simulink library "xbsDSP_r4"  (Simulink 7.1)
PreLoadFcn:
  | warning('off','MATLAB:mex:deprecatedExtension');xlmeta;com.xilinx.sysgen.util.StrategyUtil.loadAllStrategyNames();
undefined symbols (not defined in the file or in its folder): A, A2, B, C, D, gcbh, X, xlBlockLoadCallback, xlipgetpartsetting, Z
libraries: xbsIndex_r4 x27
settings Model: Tag=SysGenIndex  Creator=sysgengroup  LastModifiedBy=sysgengroup

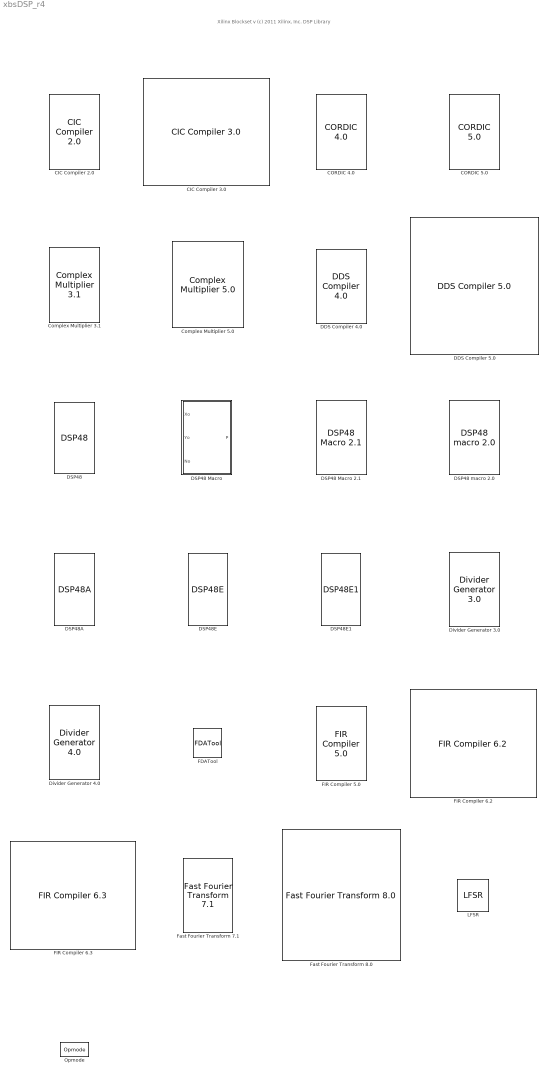
== system xbsDSP_r4 ==
  note: Xilinx Blockset v
      | (c) 2011 Xilinx, Inc.
      |
      | DSP Library
  "CIC Compiler 2.0 " : xbsIndex_r4/CIC Compiler 2.0   filter_type=Interpolation  number_of_stages=3  differential_delay=1  number_of_channels=1  sample_rate_changes=Fixed  fixed_or_initial_rate=4  minimum_rate=4  maximum_rate=4  ratespecification=Maximum_Possible  sampleperiod=4  hardwareoversamplingrate=1  quantization=Full_Precision  output_data_width=18  use_xtreme_dsp_slice=on  use_streaming_interface=on  sclr=off  ce=off  gui_behaviour=Sysgen  input_data_width=18  ip_name=CIC Compiler  ip_version=2.0  dsptool_ready=true  wrapper_available=true  port_translation_map={ 'ce' => 'en', 'sclr' => 'rst' }  ipcore_xco_need_fpga_part=true  ipcore_fpga_part=xlipgetpartsetting(gcb, {'virtex4', 'xc4vsx35', '-10', 'ff668'})  ipcore_verbose=false  block_type=cic_compiler_v2_0
  "CIC Compiler 3.0 " : xbsIndex_r4/CIC Compiler 3.0   filter_type=Interpolation  number_of_stages=3  differential_delay=1  number_of_channels=1  sample_rate_changes=Fixed  fixed_or_initial_rate=4  minimum_rate=4  maximum_rate=4  ratespecification=Maximum_Possible  sampleperiod=4  hardwareoversamplingrate=1  quantization=Full_Precision  output_data_width=22  use_xtreme_dsp_slice=on  use_streaming_interface=on  has_aclken=off  has_aresetn=off  has_dout_tready=off  trim_axipin_name=on  gui_behaviour=Sysgen_GUI  input_data_width=18  ip_name=CIC Compiler  ip_version=3.0  dsptool_ready=true  wrapper_available=true  port_translation_map={ 'aclken' => 'en', 'aresetn' => 'rst' }  ipcore_xco_need_fpga_part=true  ipcore_fpga_part=xlipgetpartsetting(gcb, {'virtex7', 'xc7v1500t', '-2', 'fhg1157'})  ipcore_verbose=false  block_type=cic_compiler_v3_0
  "CORDIC 4.0 " : xbsIndex_r4/CORDIC 4.0   functional_selection=Square_Root  architectural_configuration=Parallel  pipelining_mode=Maximum  data_format=UnsignedFraction  phase_format=Radians  output_width=16  round_mode=Truncate  iterations=0  precision=0  coarse_rotation=on  compensation_scaling=No_Scale_Compensation  ce=off  sclr=off  nd=off  rdy=off  x_out=on  y_out=on  phase_output=off  register_inputs=true  register_outputs=true  ipcore_usecache=true  ipcore_useipmodelcache=true  ipcore_verbose=false  wrapper_available=true  ip_name=CORDIC  ip_version=4.0  dsptool_ready=true  port_translation_map={ 'ce' => 'en', 'sclr' => 'rst' }  structural_sim=false  block_type=cordic_v4_0
  "CORDIC 5.0 " : xbsIndex_r4/CORDIC 5.0   functional_selection=Rotate  architectural_configuration=Parallel  pipelining_mode=Maximum  data_format=SignedFraction  phase_format=Radians  input_width=16  output_width=16  round_mode=Truncate  iterations=0  precision=0  compensation_scaling=No_Scale_Compensation  coarse_rotation=on  aclken=off  aresetn=off  out_tready=off  cartesian_has_tuser=off  cartesian_has_tlast=off  cartesian_tuser_width=1  phase_has_tuser=off  phase_has_tlast=off  phase_tuser_width=1  out_tlast_behv=Null  flow_control=NonBlocking  optimize_goal=Resources  trim_axipin_name=on  ip_name=CORDIC  ip_version=5.0  dsptool_ready=true  ipcore_usecache=true  ipcore_useipmodelcache=true  wrapper_available=true  port_translation_map={ 'aclken' => 'en', 'aresetn' => 'rst' }  block_type=cordic_v5_0
      settings: infoedit=CORDIC 5.0
  "Complex Multiplier 3.1 " : xbsIndex_r4/Complex Multiplier 3.1   multtype=Use_Mults  optimizegoal=Resources  outputwidthhigh=32  outputwidthlow=0  latency=-1  roundmode=Truncate  clockenable=off  syncclear=off  ip_name=Complex Multiplier  ip_version=3.1  dsptool_ready=true  ipcore_usecache=true  ipcore_useipmodelcache=true  ipcore_verbose=false  ipcore_latency_parameter='latency'  wrapper_available=true  port_translation_map={ 'ce' => 'en', 'sclr' => 'rst' }  structural_sim=false  block_type=cmpy_v3_1
  "Complex Multiplier 5.0 " : xbsIndex_r4/Complex Multiplier 5.0   hasatlast=off  hasatuser=off  atuserwidth=1  hasbtlast=off  hasbtuser=off  btuserwidth=1  multtype=Use_Mults  optimizegoal=Resources  flowcontrol=NonBlocking  outputwidth=33  roundmode=Truncate  hasctrltlast=off  hasctrltuser=off  ctrltuserwidth=1  outtlastbehv=Null  latencyconfig=Automatic  minimumlatency=15  aclken=off  aresetn=off  trim_axipin_name=on  aportwidth=63  bportwidth=63  ip_name=Complex Multiplier  ip_version=5.0  dsptool_ready=true  ipcore_usecache=true  ipcore_useipmodelcache=true  ipcore_verbose=false  ipcore_latency_parameter='minimumlatency'  wrapper_available=true  port_translation_map={ 'aclken' => 'en', 'aresetn' => 'rst'}  structural_sim=false  block_type=cmpy_v5_0
  "DDS Compiler 4.0 " : xbsIndex_r4/DDS Compiler 4.0   partspresent=Phase_Generator_and_SIN_COS_LUT  dds_clock_rate=100  channels=1  parameter_entry=System_Parameters  spurious_free_dynamic_range=36  frequency_resolution=0.4  noise_shaping=None  phase_width=28  output_width=6  output_selection=Sine_and_Cosine  negative_sine=off  negative_cosine=off  amplitude_mode=Full_Range  memory_type=Auto  optimization_goal=Auto  dsp48_use=Minimal  latency_configuration=Auto  latency=1  has_phase_out=on  sclr_pin=off  clock_enable=off  rfd=off  rdy=off  channel_pin=off  explicit_period=off  period=1  phase_increment=Fixed  output_frequency1=0  output_frequency2=0  output_frequency3=0  output_frequency4=0  output_frequency5=0  output_frequency6=0  output_frequency7=0  output_frequency8=0  output_frequency9=0  output_frequency10=0  output_frequency11=0  output_frequency12=0  output_frequency13=0  output_frequency14=0  output_frequency15=0  output_frequency16=0  pinc1='0'  pinc2='0'  pinc3='0'  pinc4='0'  pinc5='0'  pinc6='0'  pinc7='0'  pinc8='0'  pinc9='0'  pinc10='0'  pinc11='0'  pinc12='0'  pinc13='0'  pinc14='0'  pinc15='0'  pinc16='0'  phase_offset=None  phase_offset_angles1=0  phase_offset_angles2=0  phase_offset_angles3=0  phase_offset_angles4=0  phase_offset_angles5=0  phase_offset_angles6=0  phase_offset_angles7=0  phase_offset_angles8=0  phase_offset_angles9=0  phase_offset_angles10=0  phase_offset_angles11=0  phase_offset_angles12=0  phase_offset_angles13=0  phase_offset_angles14=0  phase_offset_angles15=0  phase_offset_angles16=0  poff1='0'  poff2='0'  poff3='0'  poff4='0'  poff5='0'  poff6='0'  poff7='0'  poff8='0'  poff9='0'  poff10='0'  poff11='0'  poff12='0'  poff13='0'  poff14='0'  poff15='0'  poff16='0'  por_mode=false  gui_behaviour=Sysgen  ip_name=DDS Compiler  ip_version=4.0  dsptool_ready=true  wrapper_available=true  port_translation_map={ 'ce' => 'en', 'sclr' => 'rst' }  ipcore_xco_need_fpga_part=true  ipcore_fpga_part=xlipgetpartsetting(gcb, {'virtex4', 'xc4vsx35', '-10', 'ff668'})  ipcore_usecache=true  ipcore_useipmodelcache=true  ipcore_verbose=false  block_type=dds_compiler_v4_0
  "DDS Compiler 5.0 " : xbsIndex_r4/DDS Compiler 5.0   partspresent=Phase_Generator_and_SIN_COS_LUT  dds_clock_rate=100  channels=1  parameter_entry=System_Parameters  spurious_free_dynamic_range=36  frequency_resolution=0.4  noise_shaping=None  phase_width=28  output_width=6  output_selection=Sine_and_Cosine  negative_sine=off  negative_cosine=off  amplitude_mode=Full_Range  memory_type=Auto  optimization_goal=Auto  dsp48_use=Minimal  latency_configuration=Auto  latency=1  has_phase_out=on  has_aclken=off  has_aresetn=off  explicit_period=off  period=1  data_has_tlast=Not_Required  has_tready=on  s_phase_has_tuser=Not_Required  m_data_has_tuser=Not_Required  m_phase_has_tuser=Not_Required  s_phase_tuser_width=1  s_config_sync_mode=On_Vector  phase_increment=Fixed  output_frequency1=0  output_frequency2=0  output_frequency3=0  output_frequency4=0  output_frequency5=0  output_frequency6=0  output_frequency7=0  output_frequency8=0  output_frequency9=0  output_frequency10=0  output_frequency11=0  output_frequency12=0  output_frequency13=0  output_frequency14=0  output_frequency15=0  output_frequency16=0  pinc1='0'  pinc2='0'  pinc3='0'  pinc4='0'  pinc5='0'  pinc6='0'  pinc7='0'  pinc8='0'  pinc9='0'  pinc10='0'  pinc11='0'  pinc12='0'  pinc13='0'  pinc14='0'  pinc15='0'  pinc16='0'  phase_offset=None  phase_offset_angles1=0  phase_offset_angles2=0  phase_offset_angles3=0  phase_offset_angles4=0  phase_offset_angles5=0  phase_offset_angles6=0  phase_offset_angles7=0  phase_offset_angles8=0  phase_offset_angles9=0  phase_offset_angles10=0  phase_offset_angles11=0  phase_offset_angles12=0  phase_offset_angles13=0  phase_offset_angles14=0  phase_offset_angles15=0  phase_offset_angles16=0  poff1='0'  poff2='0'  poff3='0'  poff4='0'  poff5='0'  poff6='0'  poff7='0'  poff8='0'  poff9='0'  poff10='0'  poff11='0'  poff12='0'  poff13='0'  poff14='0'  poff15='0'  poff16='0'  trim_axipin_name=on  por_mode=false  gui_behaviour=Sysgen  ip_name=DDS Compiler  ip_version=5.0  dsptool_ready=true  wrapper_available=true  port_translation_map={ 'aclken' => 'en', 'aresetn' => 'rst' }  ipcore_xco_need_fpga_part=true  ipcore_fpga_part=xlipgetpartsetting(gcb, {'virtex6', 'xc6vlx75t', '-3', 'ff784'})  ipcore_usecache=true  ipcore_useipmodelcache=true  ipcore_verbose=false  block_type=dds_compiler_v5_0
  DSP48 : xbsIndex_r4/DSP48  use_b=Direct from B Port  use_op=off  use_creg=off  use_pcin=off  use_pcout=off  use_bcout=off  rst_all=off  en_all=off  pipeline_a=1  pipeline_b=1  pipeline_c=on  pipeline_p=on  pipeline_mult=on  pipeline_opmode=on  pipeline_sub=on  pipeline_carryin=on  pipeline_carryinsel=on  rst_a=off  rst_b=off  rst_c=off  rst_mult=off  rst_p=off  rst_carry_in=off  rst_ctrl=off  en_a=off  en_b=off  en_c=off  en_mult=off  en_p=off  en_carry_in=off  en_ctrl=off  dbl_ovrd=off  use_synth_model=off  xl_useadderonly=off  block_type=dsp48
  DSP48 Macro : Subsystem  LoadFcn=xlBlockLoadCallback(gcbh);  mask(Xilinx DSP48 Macro Block){infoedit=Macro function to simplify use of the DSP48 primitive, especially as a dynamic operator, portalist=Xo, portblist=Yo, portclist=No, instrlist=|, pipeline_sgadvanced=, pipeline=Custom, pipeachoices_sgadvanced=, pipeachoices=1, pipebchoices_sgadvanced=, pipebchoices=1, pipecchoices_sgadvanced=, pipecchoices=on, pipepchoices_sgadvanced=, pipepchoices=on, pipemchoices_sgadvanced=, pipemchoices=on, pipectrlchoices_sgadvanced=, pipectrlchoices=on, pipemuxachoices_sgadvanced=, pipemuxachoices=0, pipemuxbchoices_sgadvanced=, pipemuxbchoices=0, pipemuxcchoices_sgadvanced=, pipemuxcchoices=0, pipemuxctrlchoices_sgadvanced=, pipemuxctrlchoices=0, pipeline_array_flag_sgadvanced=, pipeline_array_flag=off, custom_pipeline_cache=[1  1  1  1  1  1  0  0  0  0], precision_sgadvanced=, precision=Full, arith_type_sgadvanced=, arith_type=Unsigned, n_bits=8, bin_pt=2, bcout_sgadvanced=, bcout=off, acout_sgadvanced=, acout=off, carryout_sgadvanced=, carryout=off, carrycascout_sgadvanced=, carrycascout=off, pcout_sgadvanced=, pcout=off, rst_all_sgadvanced=, rst_all=off, rst_a_sgadvanced=, rst_a=off, rst_b_sgadvanced=, rst_b=off, rst_c_sgadvanced=, rst_c=off, rst_m_sgadvanced=, rst_m=off, rst_p_sgadvanced=, rst_p=off, rst_ctrl_sgadvanced=, rst_ctrl=off, ce_all_sgadvanced=, ce_all=off, ce_a_sgadvanced=, ce_a=off, ce_b_sgadvanced=, ce_b=off, ce_c_sgadvanced=, ce_c=off, ce_m_sgadvanced=, ce_m=off, ce_p_sgadvanced=, ce_p=off, ce_ctrl_sgadvanced=, ce_ctrl=off, dbl_ovrd_sgadvanced=, dbl_ovrd=off, synth_opt_sgadvanced=, synth_opt=on, errorlist=false, statestr=2d82c218ef9225b6e0048b8063710b3c, explicit_period=, period=1, maskdoc=, has_advanced_control=0, sggui_pos=-1,-1,-1,-1, block_type=dsp48macro, block_version=8.2.1, sg_icon_stat=90,138,3,1,white,blue,0,024d3c91cd129fc3834d91e223da5447,right,,[ ],[ ], sg_mask_display=|, sg_list_contents=, sg_blockgui_xml=}
      mask instrlist=|
      | <html><head><meta name="qrichtext" content="1" /></head><body style="font-size:8pt;font-family:MS Shell Dlg">
      | <p>P=Xo*Yo+No</p>
      | </body></html>
      mask sg_mask_display=|
      | fprintf('','COMMENT: begin icon graphics');
      | patch([0 90 90 0 0 ],[0 0 138 138 0 ],[0.77 0.82 0.91 ]);
      | plot([0 90 90 0 0 ],[0 0 138 138 0 ]);
      | patch([18.3 35.64 47.64 59.64 71.64 47.64 30.3 18.3 ],[82.32 82.32 94.32 82.32 94.32 94.32 94.32 82.32 ],[1 1 1 ]);
      | patch([30.3 47.64 35.64 18.3 30.3 ],[70.32 70.32 82.32 82.32 70.32 ],[0.931 0.946 0.973 ]);
      | patch([18.3 35.64 47.64 30.3 18.3 ],[58.32 58.32 70.32 70.32 58.32 ],[1 1 1 ]);
      | patch([30.3 71.64 59.64 47.64 35.64 18.3 30.3 ],[46.32 46.32 58.32 46.32 58.32 58.32 46.32 ],[0.931 0.946 0.973 ]);
      | fprintf('','COMMENT: end icon graphics');
      | fprintf('','COMMENT: begin icon text');
      | color('black');port_label('input',1,'Xo');
      | color('black');port_label('input',2,'Yo');
      | color('black');port_label('input',3,'No');
      | color('black');port_label('output',1,'P');
      | fprintf('','COMMENT: end icon text');
      mask prompts: infoedit ""; portalist "Inputs to port <tt>A</tt>"; portblist "Inputs to port <tt>B</tt>"; portclist "Inputs to port <tt>C</tt>"; instrlist "Instructions"; pipeline_sgadvanced ""; pipeline "Pipeline options"; pipeachoices_sgadvanced ""; pipeachoices "<tt>A</tt>"; pipebchoices_sgadvanced ""; pipebchoices "<tt>B</tt>"; pipecchoices_sgadvanced ""; pipecchoices "<tt>C</tt>"; pipepchoices_sgadvanced ""; pipepchoices "<tt>P</tt>"; pipemchoices_sgadvanced ""; pipemchoices "Multiplier"; pipectrlchoices_sgadvanced ""; pipectrlchoices "Controls (<tt>opmode</tt>, <tt>subtract</tt>,<br> <tt>carry_in</tt>, <tt>carry_in_sel</tt>)"; pipemuxachoices_sgadvanced ""; pipemuxachoices "MuxA"; pipemuxbchoices_sgadvanced ""; pipemuxbchoices "MuxB"; pipemuxcchoices_sgadvanced ""; pipemuxcchoices "MuxC"; pipemuxctrlchoices_sgadvanced ""; pipemuxctrlchoices "MuxCtrl"; pipeline_array_flag_sgadvanced ""; pipeline_array_flag "Define Using Array"; custom_pipeline_cache "Custom Pipeline Options([A,B,C,P,Ctrl,M,MuxA,MuxB,MuxC,MuxCtrl])"; precision_sgadvanced ""; arith_type_sgadvanced ""; arith_type "Output type"; n_bits "Number of bits"; bin_pt "Binary point"; bcout_sgadvanced ""; bcout "<tt>BCOUT</tt>"; acout_sgadvanced ""; acout "<tt>ACOUT</tt>"; carryout_sgadvanced ""; carryout "<tt>CARRYOUT</tt>"; carrycascout_sgadvanced ""; carrycascout "<tt>CARRYCASCOUT</tt>"; pcout_sgadvanced ""; pcout "<tt>PCOUT</tt>"; rst_all_sgadvanced ""; rst_all "<tt>Global Reset</tt>"; rst_a_sgadvanced ""; rst_a "Reset port for <tt>A</tt>"; rst_b_sgadvanced ""; rst_b "Reset port for <tt>B</tt>"; rst_c_sgadvanced ""; rst_c "Reset port for <tt>C</tt>"; rst_m_sgadvanced ""; rst_m "Reset port for multiplier"; rst_p_sgadvanced ""; rst_p "Reset port for <tt>P</tt>"; rst_ctrl_sgadvanced ""; rst_ctrl "Reset port for controls <br> (<tt>opmode</tt>, <tt>subtract</tt>,<br> <tt>carry_in</tt>, <tt>carry_in_sel</tt>)"; ce_all_sgadvanced ""; ce_all "<tt>Global Enable</tt>"; ce_a_sgadvanced ""; ce_a "Enable port for <tt>A</tt>"; ce_b_sgadvanced ""; ce_b "Enable port for <tt>B</tt>"; ce_c_sgadvanced ""; ce_c "Enable port for <tt>C</tt>"; ce_m_sgadvanced ""; ce_m "Enable port for multiplier"; ce_p_sgadvanced ""; ce_p "Enable port for <tt>P</tt>"; ce_ctrl_sgadvanced ""; ce_ctrl "Enable port for controls <br> (<tt>opmode</tt>, <tt>subtract</tt>,<br> <tt>carry_in</tt>, <tt>carry_in_sel</tt>)"; dbl_ovrd_sgadvanced ""; dbl_ovrd "Override with doubles"; synth_opt_sgadvanced ""; synth_opt "Use DSP48"; errorlist ""; statestr ""; explicit_period ""; period ""; maskdoc ""; has_advanced_control ""; sggui_pos ""; block_type ""; block_version ""; sg_icon_stat ""; sg_mask_display ""; sg_list_contents ""; sg_blockgui_xml ""
      mask help: Macro function to simplify use of the DSP48 primitive, especially as a dynamic operator
      mask init:
      | try
      |   tmp_gcb = gcb;
      |   tmp_gcbh = gcbh;
      |   if (strcmp('SysGenIndex',get_param(bdroot(tmp_gcbh),'tag')) && ~isempty(regexp(bdroot(tmp_gcb), '^xbs', 'once')))
      |     return;
      |   end;
      |   xlMungeMaskParams;
      | 
      |   block_type='dsp48macro';
      | 
      |   serialized_declarations = '{''block_type''=>''String''}';
      |   xldsp48macro_init();
      |   ptable_ = xlblockprep(get_param(tmp_gcb, 'MaskWSVariables'));
      |   try
      |     xlBlockMoveCallback(tmp_gcbh);
      |   catch 
      |      clear global xl_updateicon_recursion_guard;
      |   end;
      | catch
      |   global dbgsysgen;
      |   if(~isempty(dbgsysgen) && dbgsysgen)
      |     e = regexprep(lasterr, '\n', '\nError: ');
      |     disp(['Error: While running MaskInit code on block ' tmp_gcb ': ' e]);
      |     error(e);
      |   end
      | end
      settings: CopyFcn=tmp_gcbh = gcbh;set_param(tmp_gcbh,'linkstatus','none');xlBlockMoveCallback(gcbh);  DeleteFcn=xlDestroyGui(gcbh);  ModelCloseFcn=xlDestroyGui(gcbh);  PreSaveFcn=xlBlockPreSaveCallback(gcbh);  PostSaveFcn=xlBlockPostSaveCallback(gcbh);  DestroyFcn=xlDestroyGui(gcbh);  OpenFcn=xlOpenGui(gcbh, 'dsp48macro_gui.xml', @dsp48macroenablement, @dsp48macroaction)  CloseFcn=xlDestroyGui(gcbh);  MoveFcn=xlBlockMoveCallback(gcbh);
      mask Help: eval('');xlDoc('-book','sysgen','-topic','DSP48_Macro');
      mask StyleString: edit,edit,edit,edit,edit,edit,popup(External Registers|No External Registers|Custom),edit,popup(0|1|2),edit,popup(0|1|2),edit,checkbox,edit,checkbox,edit,checkbox,edit,checkbox,edit,popup(0|1|2),edit,popup(0|1|2),edit,popup(0|1|2),edit,popup(0|1|2),edit,checkbox,edit,edit,popup(Full|User Defined),edit,popup(Signed  (2's comp)|Unsigned),edit,edit,edit,checkbox,edit,checkbox,edit,checkbox,edit,checkbox,edit,checkbox,edit,checkbox,edit,checkbox,edit,checkbox,edit,checkbox,edit,checkbox,edit,checkbox,edit,checkbox,edit,checkbox,edit,checkbox,edit,checkbox,edit,checkbox,edit,checkbox,edit,checkbox,edit,checkbox,edit,checkbox,edit,checkbox,edit,edit,edit,edit,edit,edit,edit,edit,edit,edit,edit,edit,edit
      mask Display:
      | fprintf('','COMMENT: begin icon graphics');
      | patch([0 90 90 0 0 ],[0 0 138 138 0 ],[0.77 0.82 0.91 ]);
      | plot([0 90 90 0 0 ],[0 0 138 138 0 ]);
      | patch([18.3 35.64 47.64 59.64 71.64 47.64 30.3 18.3 ],[82.32 82.32 94.32 82.32 94.32 94.32 94.32 82.32 ],[1 1 1 ]);
      | patch([30.3 47.64 35.64 18.3 30.3 ],[70.32 70.32 82.32 82.32 70.32 ],[0.931 0.946 0.973 ]);
      | patch([18.3 35.64 47.64 30.3 18.3 ],[58.32 58.32 70.32 70.32 58.32 ],[1 1 1 ]);
      | patch([30.3 71.64 59.64 47.64 35.64 18.3 30.3 ],[46.32 46.32 58.32 46.32 58.32 58.32 46.32 ],[0.931 0.946 0.973 ]);
      | fprintf('','COMMENT: end icon graphics');
      | fprintf('','COMMENT: begin icon text');
      | color('black');port_label('input',1,'Xo');
      | color('black');port_label('input',2,'Yo');
      | color('black');port_label('input',3,'No');
      | color('black');port_label('output',1,'P');
      | fprintf('','COMMENT: end icon text');
  "DSP48 Macro 2.1 " : xbsIndex_r4/DSP48 Macro 2.1   instruction_list=A*B+C  AvailableInstructions=A*B+C  show_filtered=off  pipeline_options=Automatic  dspimage="<html><img src=\"xbip_dsp48_macro_v2_1_regimag.png\"></html>"  tier_1=off  tier_2=off  tier_3=off  tier_4=off  tier_5=off  tier_6=off  dreg_1=off  dreg_2=off  dreg_3=off  areg_1=off  areg_2=off  areg_3=off  areg_4=off  breg_1=off  breg_2=off  breg_3=off  breg_4=off  mreg_5=off  concatreg_3=off  concatreg_4=off  concatreg_5=off  creg_1=off  creg_2=off  creg_3=off  creg_4=off  creg_5=off  preg_6=off  cinreg_1=off  cinreg_2=off  cinreg_3=off  cinreg_4=off  cinreg_5=off  opreg_1=off  opreg_2=off  opreg_3=off  opreg_4=off  opreg_5=off  output_properties=Full_Precision  p_width=48  p_binarywidth=0  has_acout=off  has_bcout=off  has_pcout=off  has_carryout=off  has_carrycascout=off  has_ce=off  has_d_ce=off  has_a_ce=off  has_b_ce=off  has_concat_ce=off  has_c_ce=off  has_m_ce=off  has_p_ce=off  has_sel_ce=off  has_sclr=off  has_d_sclr=off  has_a_sclr=off  has_b_sclr=off  has_concat_sclr=off  has_c_sclr=off  has_m_sclr=off  has_p_sclr=off  has_sel_sclr=off  use_dsp48=on  gui_behaviour=Sysgen  instruction1=#  ip_name=DSP48 Macro  ip_version=2.1  dsptool_ready=true  ipcore_usecache=true  ipcore_useipmodelcache=true  wrapper_available=true  port_translation_map={ 'ce' => 'en', 'sclr' => 'rst'}  ipcore_xco_need_fpga_part=true  ipcore_fpga_part=xlipgetpartsetting(gcb, {'virtex6', 'xc6vlx75t', '-3', 'ff784'})  ipcore_latency_function='has_combinational'  structural_sim=false  ipcore_verbose=false  ipcore_port_config={ 'carryin' => { 'arith' => 'ufix', 'binpt' => 0.00000000000, 'width' => 1.00000000000}, 'carrycascin' => { 'arith' => 'ufix', 'binpt' => 0.00000000000, 'width' => 1.00000000000}, 'carrycascout' => { 'arith' => 'ufix', 'binpt' => 0.00000000000, 'width' => 1.00000000000}, 'carryout' => { 'arith' => 'ufix', 'binpt' => 0.00000000000, 'width' => 1.00000000000}}  block_type=xbip_dsp48_macro_v2_1
      settings: infoedit=<html>Valid operands: CONCAT, P, C, PCIN, P>>17, PCIN>>17, CARRYIN, CARRYCASCIN, ACIN, A, BCIN,B<br><br>Valid operators: +, -, *, ()<br><br>Valid functions: RNDSIMPLE, RNDSYM<br><br>Instructions are case insensitive and tolerate spaces.</html>
  "DSP48 macro 2.0 " : xbsIndex_r4/DSP48 macro 2.0   instruction_list=A*B+C  AvailableInstructions=A*B+C  show_filtered=off  pipeline_options=Automatic  dspimage="<html><img src=\"xbip_dsp48_macro_v2_0_regimag.png\"></html>"  tier_1=off  tier_2=off  tier_3=off  tier_4=off  tier_5=off  tier_6=off  dreg_1=off  dreg_2=off  dreg_3=off  areg_1=off  areg_2=off  areg_3=off  areg_4=off  breg_1=off  breg_2=off  breg_3=off  breg_4=off  mreg_5=off  concatreg_3=off  concatreg_4=off  concatreg_5=off  creg_1=off  creg_2=off  creg_3=off  creg_4=off  creg_5=off  preg_6=off  cinreg_1=off  cinreg_2=off  cinreg_3=off  cinreg_4=off  cinreg_5=off  opreg_1=off  opreg_2=off  opreg_3=off  opreg_4=off  opreg_5=off  output_properties=Full_Precision  p_width=48  p_binarywidth=0  has_carryout=off  has_acout=off  has_bcout=off  has_carrycascout=off  has_pcout=off  has_ce=off  has_sclr=off  use_dsp48=on  gui_behaviour=Sysgen  instruction1=#  ip_name=DSP48 macro  ip_version=2.0  dsptool_ready=true  ipcore_usecache=true  ipcore_useipmodelcache=true  wrapper_available=true  port_translation_map={ 'ce' => 'en', 'sclr' => 'rst'}  ipcore_xco_need_fpga_part=true  ipcore_fpga_part=xlipgetpartsetting(gcb, {'virtex4', 'xc4vsx35', '-10', 'ff668'})  ipcore_latency_function='has_combinational'  structural_sim=false  ipcore_verbose=false  ipcore_port_config={ 'carryin' => { 'arith' => 'ufix', 'binpt' => 0.00000000000, 'width' => 1.00000000000}, 'carrycascin' => { 'arith' => 'ufix', 'binpt' => 0.00000000000, 'width' => 1.00000000000}, 'carrycascout' => { 'arith' => 'ufix', 'binpt' => 0.00000000000, 'width' => 1.00000000000}, 'carryout' => { 'arith' => 'ufix', 'binpt' => 0.00000000000, 'width' => 1.00000000000}}  block_type=xbip_dsp48_macro_v2_0
      settings: infoedit=<html>Valid operands: CONCAT, P, C, PCIN, P>>17, PCIN>>17, CARRYIN, CARRYCASCIN, ACIN, A, BCIN,B<br><br>Valid operators: +, -, *, ()<br><br>Valid functions: RNDSIMPLE, RNDSYM<br><br>Instructions are case insensitive and tolerate spaces.</html>
  DSP48A : xbsIndex_r4/DSP48A  use_op=on  use_creg=off  use_d=off  use_pcin=off  use_pcout=off  use_bcout=off  use_carryin=off  use_carryout=off  rst_all=off  en_all=off  carryin_type=Direct from carry in port  use_a0reg=on  use_a1reg=on  use_b0reg=on  use_b1reg=on  pipeline_c=on  pipeline_d=on  pipeline_mult=on  pipeline_p=on  pipeline_opmode=on  pipeline_carryin=on  rst_a=off  rst_b=off  rst_c=off  rst_d=off  rst_mult=off  rst_p=off  rst_opmode=off  rst_carry_in=off  en_a=off  en_b=off  en_c=off  en_d=off  en_mult=off  en_p=off  en_opmode=off  en_carry_in=off  dbl_ovrd=off  use_synth_model=off  device=3  block_type=dsp48a
  DSP48E : xbsIndex_r4/DSP48E  use_a=Direct from A Port  use_b=Direct from B Port  reset_preg=off  pattern_from_creg=on  pattern='000000000000'  mask_from_creg=on  pattern_mask='000000000000'  sel_rounding_mask=Select mask  use_op=off  use_creg=off  rst_all=off  en_all=off  use_pcin=off  use_carrycascin=off  use_multsignin=off  use_carryout=off  use_patterndetect=off  use_patternbdetect=off  use_overflow=off  use_underflow=off  use_acout=off  use_bcout=off  use_pcout=off  use_multsignout=off  use_carrycascout=off  pipeline_a=1  pipeline_b=1  pipeline_acout=1  pipeline_bcout=1  pipeline_c=on  pipeline_p=on  pipeline_mult=on  pipeline_opmode=on  pipeline_alumode=on  pipeline_carryin=on  pipeline_carryinsel=on  rst_a=off  rst_b=off  rst_c=off  rst_mult=off  rst_p=off  rst_carry_in=off  rst_alumode=off  rst_ctrl=off  en_a1=off  en_a2=off  en_b1=off  en_b2=off  en_c=off  en_mult=off  en_p=off  en_carry_in=off  en_alumode=off  en_multcarryin=off  en_ctrl=off  use_synth_model=off  addsub_mode=ONE48  xl_useadderonly=off  block_type=dsp48e
  "DSP48E1 " : xbsIndex_r4/DSP48E1   use_a=Direct from A Port  use_b=Direct from B Port  addsub_mode=ONE48  xl_useadderonly=off  xl_dynamicmult=off  enable_preadder=off  reset_preg=off  pattern_from_creg=1  pattern='000000000000'  mask_from_creg=1  pattern_mask='000000000000'  use_op=off  use_creg=off  rst_all=off  en_all=off  use_pcin=off  use_carrycascin=off  use_multsignin=off  use_carryout=off  use_patterndetect=off  use_patternbdetect=off  use_overflow=off  use_underflow=off  use_acout=off  use_bcout=off  use_pcout=off  use_multsignout=off  use_carrycascout=off  pipeline_a=1  pipeline_b=1  pipeline_acout=1  pipeline_bcout=1  pipeline_c=on  pipeline_p=on  pipeline_mult=on  pipeline_opmode=on  pipeline_alumode=on  pipeline_carryin=on  pipeline_carryinsel=on  dreg=off  adreg=off  register_inmode=off  rst_a=off  rst_b=off  rst_c=off  rst_mult=off  rst_p=off  rst_carry_in=off  rst_alumode=off  rst_ctrl=off  reset_port_d=off  reset_port_inmode=off  en_a1=off  en_a2=off  en_b1=off  en_b2=off  en_c=off  en_mult=off  en_p=off  en_carry_in=off  en_alumode=off  en_multcarryin=off  en_ctrl=off  enable_port_regd=off  enable_port_regad=off  enable_port_reginmode=off  use_synth_model=off  block_type=dsp48e1
  "Divider Generator 3.0 " : xbsIndex_r4/Divider Generator 3.0   dividend_and_quotient_width=2  divisor_width=32  algorithm_type=Radix2  remainder_type=Remainder  fractional_width=16  clocks_per_division=1  divide_by_zero_detect=off  latency_configuration=Automatic  latency=25  ce=off  sclr=off  sclr_ce_priority=CE_overrides_SCLR  operand_sign=Signed  ip_name=Divider Generator  ip_version=3.0  dsptool_ready=true  wrapper_available=true  port_translation_map={ 'ce' => 'en', 'sclr' => 'rst' }  ipcore_fpga_part=xlipgetpartsetting(gcb, {'virtex4', 'xc4vsx35', '-10', 'ff668'})  ipcore_verbose=false  block_type=div_gen_v3_0
  "Divider Generator 4.0 " : xbsIndex_r4/Divider Generator 4.0   algorithm_type=Radix2  remainder_type=Remainder  fractional_width=16  clocks_per_division=1  divide_by_zero_detect=off  flowcontrol=NonBlocking  optimizegoal=Resources  latency_configuration=Automatic  latency=20  dividend_has_tuser=off  dividend_has_tlast=off  divisor_has_tuser=off  divisor_has_tlast=off  aclken=off  aresetn=off  outtready=off  outtlastbehv=Null  trim_axipin_name=on  dividend_tuser_width=1  divisor_tuser_width=1  operand_sign=Signed  dividend_and_quotient_width=16  divisor_width=16  ip_name=Divider Generator  ip_version=4.0  dsptool_ready=true  ipcore_usecache=true  ipcore_useipmodelcache=true  wrapper_available=true  port_translation_map={'aclken' => 'en','aresetn' => 'rst'}  ipcore_fpga_part=xlipgetpartsetting(gcb, {'virtex7', 'xc7v1500t', '-2', 'fhg1157'})  ipcore_verbose=false  block_type=div_gen_v4_0
      settings: infoedit=Divider Generator 4.0
  FDATool : xbsIndex_r4/FDATool  block_type=fdatool
      settings: infoedit=FDATool
  "FIR Compiler 5.0 " : xbsIndex_r4/FIR Compiler 5.0   coefficientvector=[6,0,-4,-3,5,6,-6,-13,7,44,64,44,7,-13,-6,6,5,-3,-4,0,6]  coefficient_sets=1  filter_type=Single_Rate  rate_change_type=Integer  interpolation_rate=2  decimation_rate=1  zero_pack_factor=1  number_channels=1  ratespecification=Maximum_Possible  sampleperiod=1  hardwareoversamplingrate=1  filter_architecture=Systolic_Multiply_Accumulate  coefficient_reload=off  coefficient_structure=Inferred  coefficient_sign=Signed  quantization=Integer_Coefficients  coefficient_width=16  bestprecision=on  coefficient_fractional_bits=0  number_paths=1  output_rounding_mode=Full_Precision  output_width=24  allow_rounding_approximation=off  optimization_goal=Area  has_sclr=off  has_data_valid=off  has_nd=off  has_ce=off  usechan_in_adv=off  chan_in_adv=0  data_buffer_type=Automatic  coefficient_buffer_type=Automatic  input_buffer_type=Automatic  output_buffer_type=Automatic  preference_for_other_storage=Automatic  multi_column_support=Disabled  columnconfig='1'  inter_column_pipe_length=4  passband_min=0.0  passband_max=0.5  stopband_min=0.5  stopband_max=1.0  filter_selection=1  gui_behaviour=Sysgen  registered_output=true  data_sign=Signed  data_width=16  data_fractional_bits=0  wrapper_available=true  ip_wrap_arbitrary_binary_point=true  ip_name=FIR Compiler  ip_version=5.0  dsptool_ready=true  ipcore_usecache=true  ipcore_useipmodelcache=true  ipcore_xco_need_fpga_part=true  port_translation_map={ 'ce' => 'en', 'sclr' => 'rst' }  run_core_at_system_period=true  ipcore_fpga_part=xlipgetpartsetting(gcb, {'virtex4', 'xc4vsx35', '-10', 'ff668'})  structural_sim=false  block_type=fir_compiler_v5_0
  "FIR Compiler 6.2 " : xbsIndex_r4/FIR Compiler 6.2   coefficientvector=[6,0,-4,-3,5,6,-6,-13,7,44,64,44,7,-13,-6,6,5,-3,-4,0,6]  coefficient_sets=1  filter_type=Single_Rate  rate_change_type=Integer  interpolation_rate=1  decimation_rate=1  number_channels=1  ratespecification=Maximum_Possible  sampleperiod=1  hardwareoversamplingrate=1  filter_architecture=Systolic_Multiply_Accumulate  coefficient_reload=off  coefficient_sign=Signed  quantization=Integer_Coefficients  coefficient_width=16  bestprecision=on  coefficient_fractional_bits=0  coefficient_structure=Inferred  number_paths=1  output_rounding_mode=Full_Precision  output_width=24  optimization_goal=Area  data_has_tlast=Not_Required  m_data_has_tready=off  s_data_has_fifo=off  s_data_has_tuser=Not_Required  m_data_has_tuser=Not_Required  s_config_sync_mode=On_Vector  s_config_method=Single  num_reload_slots=1  has_aclken=off  has_aresetn=off  multi_column_support=Disabled  columnconfig='1'  inter_column_pipe_length=4  data_buffer_type=Automatic  coefficient_buffer_type=Automatic  input_buffer_type=Automatic  output_buffer_type=Automatic  preference_for_other_storage=Automatic  trim_axipin_name=on  passband_min=0.0  passband_max=0.5  stopband_min=0.5  stopband_max=1.0  filter_selection=1  gui_behaviour=Sysgen_GUI  data_sign=Signed  data_width=16  data_fractional_bits=0  wrapper_available=true  ip_wrap_arbitrary_binary_point=true  ip_name=FIR Compiler  ip_version=6.2  dsptool_ready=true  ipcore_usecache=true  ipcore_useipmodelcache=true  ipcore_xco_need_fpga_part=true  port_translation_map={ 'aclken' => 'en', 'aresetn' => 'rst' }  run_core_at_system_period=true  ipcore_fpga_part=xlipgetpartsetting(gcb, {'virtex6', 'xc6vlx75t', '-3', 'ff784'})  structural_sim=false  block_type=fir_compiler_v6_2
      settings: infoedit=Maximum Possible : Maximizes oversampling rate. Abstracted input handshake (no s_data_tvalid) and automatic rate propagation.<br>Hardware Oversampling Rate : Specifies oversampling rate relative to the input sample period. Abstracted input handshake (no s_data_tvalid) and automatic rate propagation.<br>Sample Period : Specifies absolute oversampling rate. No input handshake abstraction (exposes s_data_tvalid) and no rate propagation.
  "FIR Compiler 6.3 " : xbsIndex_r4/FIR Compiler 6.3   coefficientvector=[6,0,-4,-3,5,6,-6,-13,7,44,64,44,7,-13,-6,6,5,-3,-4,0,6]  coefficient_sets=1  coefficient_reload=off  filter_type=Single_Rate  rate_change_type=Integer  interpolation_rate=1  decimation_rate=1  zero_pack_factor=1  channel_sequence=Basic  number_channels=1  pattern_list='P4-0,P4-1,P4-2,P4-3,P4-4'  number_paths=1  ratespecification=Maximum_Possible  sampleperiod=1  hardwareoversamplingrate=1  coefficient_sign=Signed  quantization=Integer_Coefficients  coefficient_width=16  bestprecision=on  coefficient_fractional_bits=0  coefficient_structure=Inferred  output_rounding_mode=Full_Precision  output_width=24  filter_architecture=Systolic_Multiply_Accumulate  optimization_goal=Area  data_buffer_type=Automatic  coefficient_buffer_type=Automatic  input_buffer_type=Automatic  output_buffer_type=Automatic  preference_for_other_storage=Automatic  multi_column_support=Automatic  columnconfig='1'  inter_column_pipe_length=4  data_has_tlast=Not_Required  m_data_has_tready=off  s_data_has_fifo=off  s_data_has_tuser=Not_Required  m_data_has_tuser=Not_Required  s_config_sync_mode=On_Vector  s_config_method=Single  num_reload_slots=1  has_aclken=off  has_aresetn=off  infoeditControl=ARESETn must be asserted for a minmum of 2 cycles  trim_axipin_name=on  passband_min=0.0  passband_max=0.5  stopband_min=0.5  stopband_max=1.0  filter_selection=1  gui_behaviour=Sysgen_GUI  data_sign=Signed  data_width=16  data_fractional_bits=0  data_tuser_width=1  wrapper_available=true  ip_wrap_arbitrary_binary_point=true  simulation_type=external_xfix  simulation_model=firv6_3_CModel:firv6_3_cmodel  ip_name=FIR Compiler  ip_version=6.3  dsptool_ready=true  ipcore_usecache=true  ipcore_useipmodelcache=true  ipcore_xco_need_fpga_part=true  port_translation_map={ 'aclken' => 'en', 'aresetn' => 'rst' }  run_core_at_system_period=true  ipcore_fpga_part=xlipgetpartsetting(gcb, {'virtex6', 'xc6vlx75t', '-3', 'ff784'})  block_type=fir_compiler_v6_3
      settings: infoedit=Maximum Possible : Maximizes oversampling rate. Abstracted input handshake (no s_data_tvalid) and automatic rate propagation.<br>Hardware Oversampling Rate : Specifies oversampling rate relative to the input sample period. Abstracted input handshake (no s_data_tvalid) and automatic rate propagation.<br>Sample Period : Specifies absolute oversampling rate. No input handshake abstraction (exposes s_data_tvalid) and no rate propagation.
  "Fast Fourier Transform 7.1 " : xbsIndex_r4/Fast Fourier Transform 7.1   transform_length=1024  implementation_options=pipelined_streaming_io  target_clock_frequency=250  target_data_throughput=50  run_time_configurable_transform_length=off  phase_factor_width=16  scaling_options=scaled  rounding_modes=truncation  output_ordering=bit_reversed_order  cyclic_prefix_insertion=off  ce=off  sclr=off  ovflo=off  input_data_offset=no_offset  memory_options_data=block_ram  memory_options_phase_factors=block_ram  number_of_stages_using_block_ram_for_data_and_phase_factors=1  memory_options_reorder=block_ram  memory_options_hybrid=off  complex_mult_type=use_mults_resources  butterfly_type=use_luts  channels=1  input_ordering=natural_order  input_width=16  simulation_type=external_xfix  simulation_model=fftv71_CModel:fftv71_cmodel  ip_name=Fast Fourier Transform  ip_version=7.1  dsptool_ready=true  wrapper_available=true  port_translation_map={ 'ce' => 'en', 'sclr' => 'rst' }  ipcore_fpga_part=xlipgetpartsetting(gcb, {'virtex4', 'xc4vsx35', '-10', 'ff668'})  block_type=xfft_v7_1
  "Fast Fourier Transform 8.0 " : xbsIndex_r4/Fast Fourier Transform 8.0   transform_length=1024  target_clock_frequency=250  target_data_throughput=50  implementation_options=pipelined_streaming_io  run_time_configurable_transform_length=off  phase_factor_width=16  scaling_options=scaled  rounding_modes=truncation  aclken=off  aresetn=off  cyclic_prefix_insertion=off  output_ordering=bit_reversed_order  throttle_scheme=nonrealtime  xk_index=off  ovflo=off  trim_axipin_name=on  memory_options_data=block_ram  memory_options_phase_factors=block_ram  number_of_stages_using_block_ram_for_data_and_phase_factors=1  memory_options_reorder=block_ram  memory_options_hybrid=off  complex_mult_type=use_mults_resources  butterfly_type=use_luts  channels=1  input_ordering=natural_order  input_width=16  simulation_model=fftv8_CModel:fftv8_cmodel  ip_name=Fast Fourier Transform  ip_version=8.0  dsptool_ready=true  ipcore_usecache=true  ipcore_useipmodelcache=true  wrapper_available=true  port_translation_map={ 'aclken' => 'en', 'aresetn' => 'rst'}  block_type=xfft_v8_0
  LFSR : xbsIndex_r4/LFSR  lfsr_type=Fibonacci  gate_type=XOR  n_bits=6  polynomial='11'  rst_value='3F'  rst=off  en=off  reloadable_seed=off  input_type=off  output_type=off  arith_type="Signed  (2's comp)"  bin_pt=4  dbl_ovrd=off  explicit_period=off  period=1  block_type=lfsr
  Opmode : xbsIndex_r4/Opmode  device=DSP48E  equ=P=C  operation=C  inmode_0_3=D+A2  inmode_4=B2  logicinstr=X + Z  z_mux=PCIN>>17  operand=+  xy_mux=P  x_mux=P  carry=CIN  dbl_ovrd=off  block_type=opmode

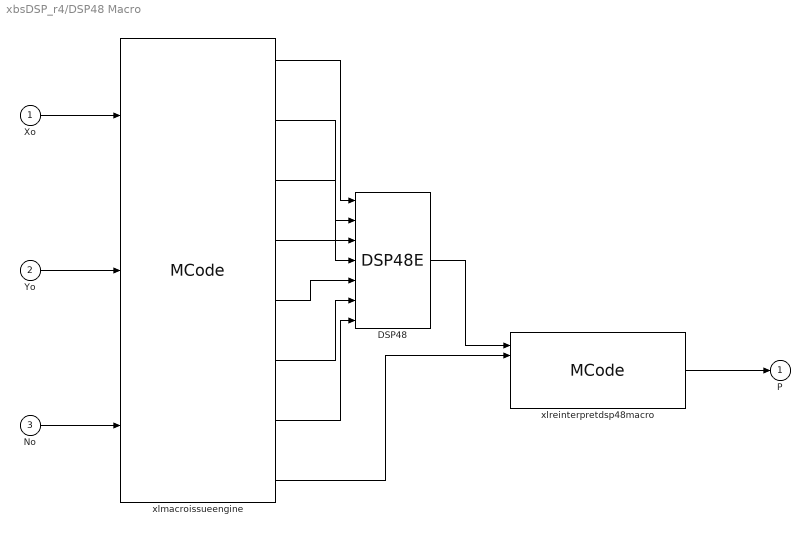
== system xbsDSP_r4/DSP48 Macro ==
  Xo : Inport  OutDataType=sfix(16)  OutScaling=2^0
  Yo : Inport  Port=2  OutDataType=sfix(16)  OutScaling=2^0
  No : Inport  Port=3  OutDataType=sfix(16)  OutScaling=2^0
  DSP48 : xbsIndex_r4/DSP48E  use_a=Direct from A Port  use_b=Direct from B Port  reset_preg=off  pattern_from_creg=on  pattern='000000000000'  mask_from_creg=on  pattern_mask='000000000000'  sel_rounding_mask=Select mask  use_op=off  use_creg=on  rst_all=off  en_all=off  use_pcin=off  use_carrycascin=off  use_multsignin=off  use_carryout=off  use_patterndetect=off  use_patternbdetect=off  use_overflow=off  use_underflow=off  use_acout=off  use_bcout=off  use_pcout=off  use_multsignout=off  use_carrycascout=off  pipeline_a=1  pipeline_b=1  pipeline_acout=1  pipeline_bcout=1  pipeline_c=on  pipeline_p=on  pipeline_mult=on  pipeline_opmode=on  pipeline_alumode=on  pipeline_carryin=on  pipeline_carryinsel=on  rst_a=off  rst_b=off  rst_c=off  rst_mult=off  rst_p=off  rst_carry_in=off  rst_alumode=off  rst_ctrl=off  en_a1=off  en_a2=off  en_b1=off  en_b2=off  en_c=off  en_mult=off  en_p=off  en_carry_in=off  en_alumode=off  en_multcarryin=off  en_ctrl=off  use_synth_model=off  addsub_mode=ONE48  xl_useadderonly=off  block_type=dsp48e
  xlmacroissueengine : xbsIndex_r4/MCode  mfname=xlissue_engine_v5  explicit_period=off  period=1  dbl_ovrd=off  enable_stdout=off  enable_debug=off  suppress_output=on  defparams={'id_a1', 0,'id_a2', 0,'id_a3', 0,'id_a4', 0,'id_a5', 0,'id_a6', 0,'id_a7', 0,'id_b1', 0,'id_b2', 0,'id_b3', 0,'id_b4', 0,'id_b5', 0,'id_b6', 0,'id_b7', 0,'id_c1', 0,'id_c2', 0,'id_c3', 0,'id_c4', 0,'id_c5', 0,'id_c6', 0,'id_c7', 0,'op_const0',53,'op_const1', 0,'op_const2', 0,'op_const3', 0,'op_const4', 0,'op_const5', 0,'op_const6', 0,'op_const7', 0,'alumode_const0',0,'alumode_const1', 0,'alumode_const2', 0,'alumode_const3', 0,'alumode_const4', 0,'alumode_const5', 0,'alumode_const6', 0,'alumode_const7', 0,'carry_in_sel0',0,'carry_in_sel1', 0,'carry_in_sel2', 0,'carry_in_sel3', 0,'carry_in_sel4', 0,'carry_in_sel5', 0,'carry_in_sel6', 0,'carry_in_sel7', 0,'external_cin0', 0,'external_cin1', 0,'external_cin2', 0,'external_cin3', 0,'external_cin4', 0,'external_cin5', 0,'external_cin6', 0,'external_cin7', 0,'reg_a',0,'reg_b',0,'reg_c',0,'reg_op',0,'mode0', 1,'mode1', 0,'mode2', 0,'mode3', 0,'mode4', 0,'mode5', 0,'mode6', 0,'mode7', 0,'ce_all',true,'use_ce_all',false,'sel',0,'rst_all',false,'use_rst_all',false,'cinused',false,'ninstr',1}  hide_port_list={}  block_type=mcode
      settings: xl_area=[0, 0, 0, 0, 0, 0, 0]
  xlreinterpretdsp48macro : xbsIndex_r4/MCode  mfname=xlreinterpretdsp48macro  explicit_period=off  period=1  dbl_ovrd=off  enable_stdout=off  enable_debug=off  suppress_output=off  defparams={'full',precision,'n_bits',n_bits,'bin_pt',bin_pt,'arith_type',arith_type}  hide_port_list={}  block_type=mcode
      settings: xl_area=[0, 0, 0, 0, 0, 0, 0]
  P : Outport  OutDataType=sfix(16)  OutScaling=2^0
  wires:
  Xo/1 -> xlmacroissueengine/1
  Yo/1 -> xlmacroissueengine/2
  No/1 -> xlmacroissueengine/3
  xlmacroissueengine/1 -> DSP48/1
  xlmacroissueengine/2 -> DSP48/2
  xlmacroissueengine/3 -> DSP48/3
  xlmacroissueengine/4 -> DSP48/4
  xlmacroissueengine/5 -> DSP48/5
  xlmacroissueengine/6 -> DSP48/6
  xlmacroissueengine/7 -> DSP48/7
  xlmacroissueengine/8 -> xlreinterpretdsp48macro/2
  DSP48/1 -> xlreinterpretdsp48macro/1
  xlreinterpretdsp48macro/1 -> P/1
